simulink model "Model"  (R2024b)
settings: Solver=VariableStepAuto  StartTime=0.0  StopTime=30  MaxStep=0.001  RelTol=1e-4
PostLoadFcn:
  | SIM_setup
values from neighbouring files (symbols this model uses):
  A = 1.1    [RT14e_Parameters.m]    (also in RT15e_Parameters.m = 1.088; RT15evo_Parameters.m = 1.088; SIM_setup.m = 1.12)
  Aero_balance = 55    [RT14e_Parameters.m]    (also in RT15e_Parameters.m; RT15evo_Parameters.m; SIM_setup.m = 0.55)
  air_density = 1.29    [SIM_setup.m]
  Br_coef_of_friction_F = 0.33    [RT14e_Parameters.m]    (also in RT15e_Parameters.m; RT15evo_Parameters.m; SIM_setup.m = 0.25)
  Br_coef_of_friction_R = 0.33    [RT14e_Parameters.m]    (also in RT15e_Parameters.m; RT15evo_Parameters.m; SIM_setup.m = 0.25)
  Br_pistons_area_F = 3617.26/1e6    (= 0.00361726)    [RT14e_Parameters.m]    (also in RT15e_Parameters.m; RT15evo_Parameters.m; SIM_setup.m)
  Br_pistons_area_R = 2026.83/1e6    (= 0.00202683)    [RT14e_Parameters.m]    (also in RT15e_Parameters.m; RT15evo_Parameters.m; SIM_setup.m)
  Cd = 1.387    [SIM_setup.m]
  Cl = 3.299    [SIM_setup.m]
  CoG_z = 0.35    [RT14e_Parameters.m]    (also in RT15e_Parameters.m = 0.28495; RT15evo_Parameters.m = 0.28495; SIM_setup.m = 0.328)
  Default_Fz_F = g*(Mass*(Lr/Wheelbase))    [RT14e_Parameters.m]    (also in RT15e_Parameters.m; RT15evo_Parameters.m; SIM_setup.m = 608.22)
  Default_Fz_R = g*(Mass*(Lf/Wheelbase))    [RT14e_Parameters.m]    (also in RT15e_Parameters.m; RT15evo_Parameters.m; SIM_setup.m = 774.99)
  Effective_br_disk_r_F = 0.0905    [RT14e_Parameters.m]    (also in RT15e_Parameters.m; RT15evo_Parameters.m; SIM_setup.m)
  Effective_br_disk_r_R = 0.0895    [RT14e_Parameters.m]    (also in RT15e_Parameters.m; RT15evo_Parameters.m; SIM_setup.m)
  Fx = Data_Fx(2:end,3:end)    [RT14e_Parameters.m]    (also in RT15e_Parameters.m; RT15evo_Parameters.m; SIM_setup.m = Data_Fx(2:end,2:end))
  Fy = Data_Fy(2:end,3:end)    [RT14e_Parameters.m]    (also in RT15e_Parameters.m; RT15evo_Parameters.m; SIM_setup.m = Data_Fy(2:end,2:end))
  Fz = Data_Fy(2:end,2)    [RT14e_Parameters.m]    (also in RT15e_Parameters.m; RT15evo_Parameters.m; SIM_setup.m = Data_Fy(2:end,1))
  Half_track = 0.6    [SIM_setup.m]
  Iz_wehicle = 120    [RT14e_Parameters.m]    (also in RT15e_Parameters.m; RT15evo_Parameters.m; SIM_setup.m)
  Iz_wheel = 0.15    [RT14e_Parameters.m]    (also in RT15e_Parameters.m; RT15evo_Parameters.m; SIM_setup.m)
  Lateral_load_transfer_distribution = 0.55    [SIM_setup.m]
  Lf = Wheelbase - CoG_x    (= 0.77)    [RT14e_Parameters.m]    (also in RT15e_Parameters.m = 0.7504; RT15evo_Parameters.m = 0.7504; SIM_setup.m)
  Lr = Wheelbase - Lf    (= 0.755)    [RT14e_Parameters.m]    (also in RT15e_Parameters.m = 0.7746; RT15evo_Parameters.m = 0.7746; SIM_setup.m)
  Mass = Vehicle_mass + Driver_mass    (= 290)    [RT14e_Parameters.m]    (also in RT15e_Parameters.m = 265; RT15evo_Parameters.m; SIM_setup.m = 300)
  Max_Torque = 29.1    [SIM_setup.m]
  RB_torque_setting_1 = -2    [RT14e_Parameters.m]    (also in RT15e_Parameters.m; RT15evo_Parameters.m; SIM_setup.m)
  RB_torque_setting_10 = -20    [RT14e_Parameters.m]    (also in RT15e_Parameters.m; RT15evo_Parameters.m; SIM_setup.m)
  RB_torque_setting_2 = -4    [RT14e_Parameters.m]    (also in RT15e_Parameters.m; RT15evo_Parameters.m; SIM_setup.m)
  RB_torque_setting_3 = -6    [RT14e_Parameters.m]    (also in RT15e_Parameters.m; RT15evo_Parameters.m; SIM_setup.m)
  RB_torque_setting_4 = -8    [RT14e_Parameters.m]    (also in RT15e_Parameters.m; RT15evo_Parameters.m; SIM_setup.m)
  RB_torque_setting_5 = -10    [RT14e_Parameters.m]    (also in RT15e_Parameters.m; RT15evo_Parameters.m; SIM_setup.m)
  RB_torque_setting_6 = -12    [RT14e_Parameters.m]    (also in RT15e_Parameters.m; RT15evo_Parameters.m; SIM_setup.m)
  RB_torque_setting_7 = -14    [RT14e_Parameters.m]    (also in RT15e_Parameters.m; RT15evo_Parameters.m; SIM_setup.m)
  RB_torque_setting_8 = -16    [RT14e_Parameters.m]    (also in RT15e_Parameters.m; RT15evo_Parameters.m; SIM_setup.m)
  RB_torque_setting_9 = -18    [RT14e_Parameters.m]    (also in RT15e_Parameters.m; RT15evo_Parameters.m; SIM_setup.m)
  SA = Data_Fy(1,3:end)    [RT14e_Parameters.m]    (also in RT15e_Parameters.m; RT15evo_Parameters.m; SIM_setup.m = Data_Fy(1,2:end))
  SR = Data_Fx(1,3:end)    [RT14e_Parameters.m]    (also in RT15e_Parameters.m; RT15evo_Parameters.m; SIM_setup.m = Data_Fx(1,2:end))
  start_time = 182    [SIM_setup.m]
  start_velocity = Xsens_MTI_670_vel.Value(find(Xsens_MTI_670_vel.Time > start_time, 1)) * 1000 / 3600    [SIM_setup.m]
  Steering_angle_table = [0 9.9 19.9 30.14 40.57 51.05 61.29 70.87 79.38 91.9]    [SIM_setup.m]
  Steering_ratio_table = [3.25 3.24 3.23 3.20 3.16 3.10 3.04 2.97 2.90 2.77]    [SIM_setup.m]
  Tire_radius = 0.203    [RT14e_Parameters.m]    (also in RT15e_Parameters.m; RT15evo_Parameters.m; SIM_setup.m)
  Torque_limit_2 = Motor_maximum_torque*0.2    (= 5.82)    [RT14e_Parameters.m]    (also in RT15e_Parameters.m; RT15evo_Parameters.m; SIM_setup.m)
  Torque_limit_3 = Motor_maximum_torque*0.3    (= 8.73)    [RT14e_Parameters.m]    (also in RT15e_Parameters.m; RT15evo_Parameters.m; SIM_setup.m)
  Torque_limit_4 = Motor_maximum_torque*0.4    (= 11.64)    [RT14e_Parameters.m]    (also in RT15e_Parameters.m; RT15evo_Parameters.m; SIM_setup.m)
  Torque_limit_5 = Motor_maximum_torque*0.5    (= 14.55)    [RT14e_Parameters.m]    (also in RT15e_Parameters.m; RT15evo_Parameters.m; SIM_setup.m)
  Torque_limit_6 = Motor_maximum_torque*0.6    (= 17.46)    [RT14e_Parameters.m]    (also in RT15e_Parameters.m; RT15evo_Parameters.m; SIM_setup.m)
  Torque_limit_7 = Motor_maximum_torque*0.7    (= 20.37)    [RT14e_Parameters.m]    (also in RT15e_Parameters.m; RT15evo_Parameters.m; SIM_setup.m)
  Torque_limit_8 = Motor_maximum_torque*0.8    (= 23.28)    [RT14e_Parameters.m]    (also in RT15e_Parameters.m; RT15evo_Parameters.m; SIM_setup.m)
  Torque_limit_9 = 29.1    [RT14e_Parameters.m]    (also in RT15e_Parameters.m; RT15evo_Parameters.m; SIM_setup.m)
  Torque_limit_max = Motor_maximum_torque    (= 29.1)    [RT14e_Parameters.m]    (also in RT15e_Parameters.m; RT15evo_Parameters.m; SIM_setup.m)
  Torque_limit_min = Motor_maximum_torque*0.1    (= 2.91)    [RT14e_Parameters.m]    (also in RT15e_Parameters.m; RT15evo_Parameters.m; SIM_setup.m)
  Transmission_gear_ratio = 12.9    [SIM_setup.m]
  TV_RB_understeer_gradient_1 = -0.5    [RT14e_Parameters.m]    (also in RT15e_Parameters.m; RT15evo_Parameters.m; SIM_setup.m)
  TV_RB_understeer_gradient_10 = 0.005    [RT14e_Parameters.m]    (also in RT15e_Parameters.m; RT15evo_Parameters.m; SIM_setup.m)
  TV_RB_understeer_gradient_2 = -0.1    [RT14e_Parameters.m]    (also in RT15e_Parameters.m; RT15evo_Parameters.m; SIM_setup.m)
  TV_RB_understeer_gradient_3 = 0.08    [RT14e_Parameters.m]    (also in RT15e_Parameters.m; RT15evo_Parameters.m; SIM_setup.m)
  TV_RB_understeer_gradient_4 = 0.06    [RT14e_Parameters.m]    (also in RT15e_Parameters.m; RT15evo_Parameters.m; SIM_setup.m)
  TV_RB_understeer_gradient_5 = 0.05    [RT14e_Parameters.m]    (also in RT15e_Parameters.m; RT15evo_Parameters.m; SIM_setup.m)
  TV_RB_understeer_gradient_6 = 0.04    [RT14e_Parameters.m]    (also in RT15e_Parameters.m; RT15evo_Parameters.m; SIM_setup.m)
  TV_RB_understeer_gradient_7 = 0.03    [RT14e_Parameters.m]    (also in RT15e_Parameters.m; RT15evo_Parameters.m; SIM_setup.m)
  TV_RB_understeer_gradient_8 = 0.02    [RT14e_Parameters.m]    (also in RT15e_Parameters.m; RT15evo_Parameters.m; SIM_setup.m)
  TV_RB_understeer_gradient_9 = 0.01    [RT14e_Parameters.m]    (also in RT15e_Parameters.m; RT15evo_Parameters.m; SIM_setup.m)
  TV_understeer_gradient_1 = -0.5    [RT14e_Parameters.m]    (also in RT15e_Parameters.m; RT15evo_Parameters.m; SIM_setup.m)
  TV_understeer_gradient_10 = 0.002    [RT14e_Parameters.m]    (also in RT15e_Parameters.m; RT15evo_Parameters.m; SIM_setup.m)
  TV_understeer_gradient_2 = -0.1    [RT14e_Parameters.m]    (also in RT15e_Parameters.m; RT15evo_Parameters.m; SIM_setup.m)
  TV_understeer_gradient_3 = 0.06    [RT14e_Parameters.m]    (also in RT15e_Parameters.m; RT15evo_Parameters.m; SIM_setup.m)
  TV_understeer_gradient_4 = 0.05    [RT14e_Parameters.m]    (also in RT15e_Parameters.m; RT15evo_Parameters.m; SIM_setup.m)
  TV_understeer_gradient_5 = 0.04    [RT14e_Parameters.m]    (also in RT15e_Parameters.m; RT15evo_Parameters.m; SIM_setup.m)
  TV_understeer_gradient_6 = 0.03    [RT14e_Parameters.m]    (also in RT15e_Parameters.m; RT15evo_Parameters.m; SIM_setup.m)
  TV_understeer_gradient_7 = 0.02    [RT14e_Parameters.m]    (also in RT15e_Parameters.m; RT15evo_Parameters.m; SIM_setup.m)
  TV_understeer_gradient_8 = 0.01    [RT14e_Parameters.m]    (also in RT15e_Parameters.m; RT15evo_Parameters.m; SIM_setup.m)
  TV_understeer_gradient_9 = 0.005    [RT14e_Parameters.m]    (also in RT15e_Parameters.m; RT15evo_Parameters.m; SIM_setup.m)
  Wheel_base = 1.525    [SIM_setup.m]
  Wheel_rolling_resistance = 0.055    [RT14e_Parameters.m]    (also in RT15e_Parameters.m; RT15evo_Parameters.m; SIM_setup.m)
undefined symbols (not defined in the file or in its folder): Actual_Torque_Value_RL, Actual_Torque_Value_RR, aero_balance, APPS, Brake_Pressure_Front, Brake_Pressure_Rear, lateral_load_transfer_distribution, Steering_position, tire_radius, wheel_base, Xsens_MTI_670_accX, Xsens_MTI_670_accY, Xsens_MTI_670_gyrZ, Xsens_MTI_670_vel, Xsens_Yaw_Rate__deg_s_
libraries: simulink x20, simulink_extras x7, dspstat3 x4, slpidlib x1, slrealtimeloglib x1
(part 2 of 4)

== system Model/Drivetrain/Braking_Torque/Braking_Torque_Front ==
  Brake_Pressure [bar] : Inport
  Gain : Gain  Gain=1e5
  Gain1 : Gain  Gain=Effective_br_disk_r_F
  Product : Product  Inputs=3
  coefficient of friction : Constant  Value=Br_coef_of_friction_F
  piston area : Constant  Value=Br_pistons_area_F
  Braking torque [Nm] : Outport
  wires:
  Brake_Pressure [bar]/1 -> Gain/1  "[bar]"
  Gain/1 -> Product/1  "[Pa]"
  coefficient of friction/1 -> Product/2
  piston area/1 -> Product/3
  Product/1 -> Gain1/1  "Braking force [N]"
  Gain1/1 -> Braking torque [Nm]/1  "Braking torque [Nm]"

== system Model/Drivetrain/Braking_Torque/Braking_Torque_Rear ==
  Brake_Pressure [bar] : Inport
  Gain1 : Gain  Gain=1e5
  Gain2 : Gain  Gain=Effective_br_disk_r_R
  Product2 : Product  Inputs=3
  coefficient of friction : Constant  Value=Br_coef_of_friction_R
  piston area : Constant  Value=Br_pistons_area_R
  Braking_Torque [Nm] : Outport
  wires:
  Product2/1 -> Gain2/1  "Braking_Force [N]"
  piston area/1 -> Product2/3
  Gain2/1 -> Braking_Torque [Nm]/1  "Braking_Torque [Nm]"
  Gain1/1 -> Product2/1  "[Pa]"
  coefficient of friction/1 -> Product2/2
  Brake_Pressure [bar]/1 -> Gain1/1

== system Model/Drivetrain/Engine_Power/Engine_RL ==
  Wheel_Angular_Speed : Inport
  Engine_Torque : Inport  Port=2
  Gain : Gain  Gain=60/2*pi
  Gain1 : Gain  Gain=1/3.6e7
  Integrator : Integrator
  Product : Product
  Energy Used [kWh] : Outport
  wires:
  Gain/1 -> Product/1  "Wheel_Angular_Speed [rot/min]"
  Gain1/1 -> Energy Used [kWh]/1  "Energy_Used [kWh]"
  Integrator/1 -> Gain1/1  "Energy [J]"
  Product/1 -> Integrator/1  "Motor_Power [W]"
  Wheel_Angular_Speed/1 -> Gain/1
  Engine_Torque/1 -> Product/2

== system Model/Drivetrain/Engine_Power/Engine_RR ==
  Wheel_Angular_Speed : Inport
  Engine_Torque : Inport  Port=2
  Gain : Gain  Gain=60/2*pi
  Gain1 : Gain  Gain=1/3.6e7
  Integrator : Integrator
  Product : Product
  Energy Used [kWh] : Outport
  wires:
  Gain/1 -> Product/1  "Wheel_Angular_Speed [rot/min]"
  Gain1/1 -> Energy Used [kWh]/1  "Energy_Used [kWh]"
  Integrator/1 -> Gain1/1  "Energy [J]"
  Product/1 -> Integrator/1  "Motor_Power [W]"
  Wheel_Angular_Speed/1 -> Gain/1
  Engine_Torque/1 -> Product/2

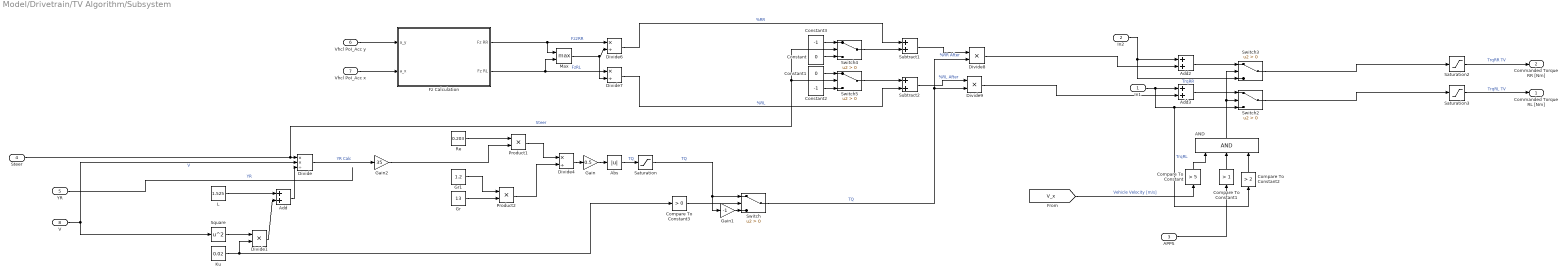
== system Model/Drivetrain/TV Algorithm/Subsystem ==
  In1 : Inport
  In2 : Inport  Port=2
  APPS : Inport  Port=3
  Steer : Inport  Port=4
  YR : Inport  Port=5
  Vhcl PoI_Acc y : Inport  Port=6
  Vhcl PoI_Acc x : Inport  Port=7
  V : Inport  Port=8
  AND : Logic  Inputs=3  IconShape=distinctive  AllPortsSameDT=off  OutDataTypeStr=boolean
  Abs : Abs  SaturateOnIntegerOverflow=off
  Add : Sum
  Add2 : Sum
  Add3 : Sum
  Compare To Constant : simulink/Logic and Bit Operations/Compare To Constant  relop=>  const=5  OutDataTypeStr=boolean
  Compare To Constant1 : simulink/Logic and Bit Operations/Compare To Constant  relop=>  const=1  OutDataTypeStr=boolean
  Compare To Constant2 : simulink/Logic and Bit Operations/Compare To Constant  relop=>  const=2  OutDataTypeStr=boolean
  Compare To Constant3 : simulink/Logic and Bit Operations/Compare To Constant  relop=>  const=0  OutDataTypeStr=boolean
  Constant : Constant  Value=0
  Constant1 : Constant  Value=0
  Constant2 : Constant  Value=-1
  Constant3 : Constant  Value=-1
  Divide : Product  Inputs=**/
  Divide1 : Product  Inputs=**
  Divide4 : Product  Inputs=*/
  Divide6 : Product  Inputs=*/
  Divide7 : Product  Inputs=*/
  Divide8 : Product  Inputs=**
  Divide9 : Product  Inputs=**
  Fz Calculation : Subsystem
  Gain : Gain  Gain=0.5
  Gain1 : Gain  Gain=-1
  Gain2 : Gain  Gain=35
  Gr : Constant  Value=13
  Gr1 : Constant  Value=1.2
  Ku : Constant  Value=0.02
  L : Constant  Value=1.525
  Max : MinMax  Function=max  Inputs=2
  Product1 : Product
  Product2 : Product
  Re : Constant  Value=0.203
  Saturation : Saturate  UpperLimit=8  LowerLimit=0
  Saturation2 : Saturate  UpperLimit=Max_Torque  LowerLimit=0
  Saturation3 : Saturate  UpperLimit=Max_Torque  LowerLimit=0
  Square : Math  Operator=square
  Subtract1 : Sum
  Subtract2 : Sum
  Switch{,2..5} (5 alike) : Switch  Criteria=u2 > Threshold  SaturateOnIntegerOverflow=off  InputSameDT=off
  Commanded Torque RL [Nm] : Outport
  Commanded Torque RR [Nm] : Outport  Port=2
  wires:
  Max/1 -> Divide7/2, Divide6/2
  Divide9/1 -> Add3/2
  L/1 -> Add/1
  Steer/1 -> Switch4/2, Switch5/2, Divide/1  "Steer"
  In1/1 -> Compare To Constant2/1, Switch2/3, Add3/1  "TrqRL"
  Vhcl PoI_Acc y/1 -> Fz Calculation/1(a_y)
  Divide8/1 -> Add2/2
  Divide6/1 -> Subtract1/1  "%RR"
  In2/1 -> Switch3/3, Add2/1  "TrqRR"
  Vhcl PoI_Acc x/1 -> Fz Calculation/2(a_x)
  Divide4/1 -> Gain/1
  Add3/1 -> Switch2/1
  Divide7/1 -> Subtract2/2  "%RL"
  Divide1/1 -> Add/2
  Ku/1 -> Compare To Constant3/1, Divide1/2
  Add/1 -> Divide/3
  Divide/1 -> Gain2/1  "YR Calc"
  Fz Calculation/2(Fz RL) -> Max/2, Divide7/1  "FzRL"
  Square/1 -> Divide1/1
  Saturation2/1 -> Commanded Torque RR [Nm]/1  "TrqRR TV"
  Saturation3/1 -> Commanded Torque RL [Nm]/1  "TrqRL TV"
  Re/1 -> Product1/1
  Product1/1 -> Divide4/1
  Gr/1 -> Product2/2
  Gain2/1 -> Product1/2
  Switch/1 -> Divide8/2, Divide9/2  "TQ"
  YR/1 -> ?  "YR"
  Gr1/1 -> Product2/1
  Product2/1 -> Divide4/2
  V/1 -> Square/1, Divide/2  "V"
  Gain/1 -> Abs/1
  Add2/1 -> Switch3/1
  [V_x] -> Compare To Constant/1  "Vehicle Velocity [m/s]"
  Compare To Constant/1 -> AND/1
  Compare To Constant1/1 -> AND/2
  APPS/1 -> Compare To Constant1/1
  AND/1 -> Switch2/2, Switch3/2
  Abs/1 -> Saturation/1  "TQ"
  Subtract1/1 -> Divide8/1  "%RR After"
  Subtract2/1 -> Divide9/1  "%RL After"
  Constant2/1 -> Switch5/3
  Switch4/1 -> Subtract1/2
  Switch5/1 -> Subtract2/1
  Constant/1 -> Switch4/3
  Constant1/1 -> Switch5/1
  Constant3/1 -> Switch4/1
  Compare To Constant2/1 -> AND/3
  Switch3/1 -> Saturation2/1
  Switch2/1 -> Saturation3/1
  Compare To Constant3/1 -> Switch/2
  Saturation/1 -> Switch/1, Gain1/1  "TQ"
  Gain1/1 -> Switch/3
  Fz Calculation/1(Fz RR) -> Max/1, Divide6/1  "Fz2RR"

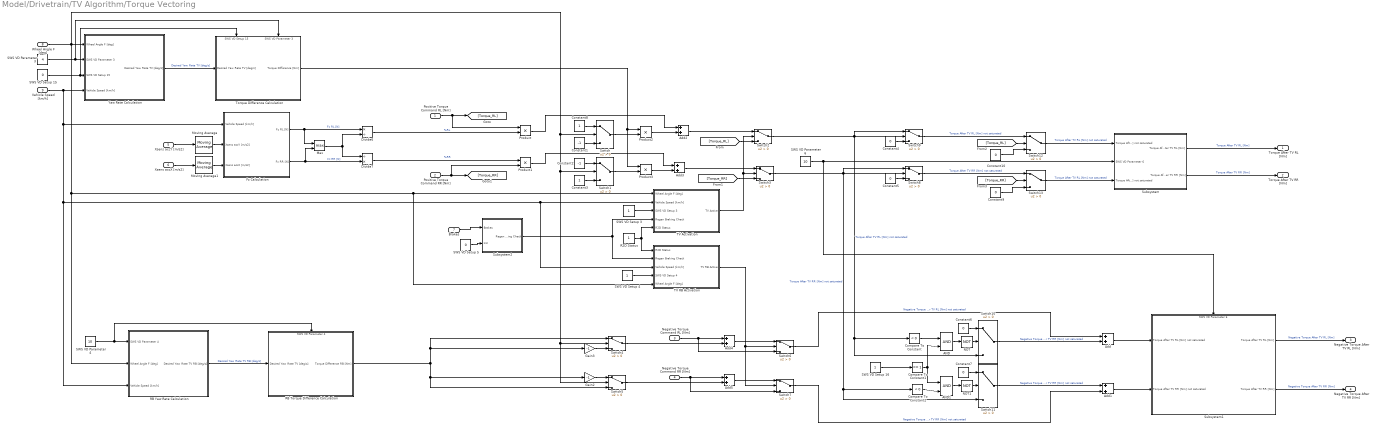
== system Model/Drivetrain/TV Algorithm/Torque Vectoring ==
  Positive Torque Command RL [Nm] : Inport
  Positive Torque Command RR [Nm] : Inport  Port=2
  Negative Torque Command RL [Nm] : Inport  Port=3
  Negative Torque Command RR [Nm] : Inport  Port=4
  Xsens accY [m/s2] : Inport  Port=5
  Xsens accX [m/s2] : Inport  Port=6
  Brakes : Inport  Port=7
  Wheel Angle F [deg] : Inport  Port=8
  Vehicle Speed [km/h] : Inport  Port=9
  AND : Logic  IconShape=distinctive  AllPortsSameDT=off  OutDataTypeStr=boolean
  AND1 : Logic  IconShape=distinctive  AllPortsSameDT=off  OutDataTypeStr=boolean
  Add{,1..5} (6 alike) : Sum
  Compare To Constant : simulink/Logic and Bit Operations/Compare To Constant  relop=<  const=0  OutDataTypeStr=boolean
  Compare To Constant1 : simulink/Logic and Bit Operations/Compare To Constant  relop===  const=1  OutDataTypeStr=boolean
  Compare To Constant2 : simulink/Logic and Bit Operations/Compare To Constant  relop=<  const=0  OutDataTypeStr=boolean
  Constant1 : Constant  Value=-1
  Constant{4..7,9..10} (6 alike) : Constant  Value=0
  Constant2 : Constant  Value=-1
  Constant3 : Constant
  Constant8 : Constant
  Divide6 : Product  Inputs=*/
  Divide7 : Product  Inputs=/*
  Fz Calculation : Subsystem
  Gain2 : Gain  Gain=-1
  Gain3 : Gain  Gain=-1
  Max : MinMax  Function=max  Inputs=2
  Moving Average : dspstat3/Moving Average  Method=Sliding window  ForgettingFactorPort=off  SpecifyWindowLength=on  WindowLength=4  OverlapLength=3  AllowArbitraryInputLength=off  ForgettingFactor=0.9  SimulateUsing=Code generation
  Moving Average1 : dspstat3/Moving Average  Method=Sliding window  ForgettingFactorPort=off  SpecifyWindowLength=on  WindowLength=4  OverlapLength=3  AllowArbitraryInputLength=off  ForgettingFactor=0.9  SimulateUsing=Code generation
  NOT : Logic  Operator=NOT  IconShape=distinctive  AllPortsSameDT=off  OutDataTypeStr=boolean
  NOT1 : Logic  Operator=NOT  IconShape=distinctive  AllPortsSameDT=off  OutDataTypeStr=boolean
  Product{,1..3} (4 alike) : Product
  R2D Status : Constant
  RB Torque Difference Calculation : Subsystem
      settings: PortSchema="{\"entries\":[{\"content\":{\"sides\":[{\"content\":{\"connectorIds\":[\"In1\"]},\"type\":\"ConnectorPlacement.EquallySpacedRectSide\",\"uuid\":\"fa4973ad-a32f-4095-ab0b-cea383016739\"},{\"content\":{\"connectorIds\":[\"Out1\"],\"side\":\"RIGHT\"},\"type\":\"ConnectorPlacement.EquallySpacedRectSide\",\"uuid\":\"939e1308-df81-4bd9-8a82-65ce288053d3\"},{\"content\":{\"connectorIds\":[\"In2\"],\"side\":\"TOP\"},\"type\":\"ConnectorPlacement.EquallySpacedRectSide\",\"uuid\":\"fc465ebf-5b67-4318-901e-ca5dd36e3a85\"}]},\"type\":\"ConnectorPlacement.EquallySpacedConnector\",\"uuid\":\"4f087700-9ed6-4341-833d-4cc93a86ad38\"}],\"packageUris\":[\"http://schema.mathworks.com/mf0/Connector/R2020b\"],\"version\":\"1.0\"}"
  RB Yaw Rate Calculation : Subsystem
  SWS VD Parameter 3 : Constant  Value=4
  SWS VD Parameter 4 : Constant  Value=10
  SWS VD Parameter 6 : Constant  Value=10
  SWS VD Setup 15 : Constant  Value=0
  SWS VD Setup 16 : Constant
  SWS VD Setup 3 : Constant
  SWS VD Setup 4 : Constant
  SWS VD Setup 5 : Constant  Value=0
  Subsystem : Subsystem
  Subsystem1 : Subsystem
      settings: PortSchema="{\"entries\":[{\"content\":{\"sides\":[{\"content\":{\"connectorIds\":[\"In1\",\"In2\"]},\"type\":\"ConnectorPlacement.EquallySpacedRectSide\",\"uuid\":\"3056adb4-125a-41ff-b8f3-94632bed0e59\"},{\"content\":{\"connectorIds\":[\"Out1\",\"Out2\"],\"side\":\"RIGHT\"},\"type\":\"ConnectorPlacement.EquallySpacedRectSide\",\"uuid\":\"828b5026-b9f0-47a0-9847-e54771aaad3f\"},{\"content\":{\"connectorIds\":[\"In3\"],\"side\":\"TOP\"},\"type\":\"ConnectorPlacement.EquallySpacedRectSide\",\"uuid\":\"5565ffc5-94d3-407e-898e-a464d97134f1\"}]},\"type\":\"ConnectorPlacement.EquallySpacedConnector\",\"uuid\":\"ef74bfd7-20f4-4a9c-8af2-e6f991f2b9d8\"}],\"packageUris\":[\"http://schema.mathworks.com/mf0/Connector/R2020b\"],\"version\":\"1.0\"}"
  Subsystem2 : Subsystem
  Switch{,1..13} (14 alike) : Switch  Criteria=u2 > Threshold  SaturateOnIntegerOverflow=off  InputSameDT=off
  TV Activation : Subsystem
  TV RB Activation : Subsystem
  Torque Difference Calculation : Subsystem
      settings: PortSchema="{\"entries\":[{\"content\":{\"sides\":[{\"content\":{\"connectorIds\":[\"In1\"]},\"type\":\"ConnectorPlacement.EquallySpacedRectSide\",\"uuid\":\"fa4973ad-a32f-4095-ab0b-cea383016739\"},{\"content\":{\"connectorIds\":[\"Out1\"],\"side\":\"RIGHT\"},\"type\":\"ConnectorPlacement.EquallySpacedRectSide\",\"uuid\":\"939e1308-df81-4bd9-8a82-65ce288053d3\"},{\"content\":{\"connectorIds\":[\"In2\",\"In3\"],\"side\":\"TOP\"},\"type\":\"ConnectorPlacement.EquallySpacedRectSide\",\"uuid\":\"fc465ebf-5b67-4318-901e-ca5dd36e3a85\"}]},\"type\":\"ConnectorPlacement.EquallySpacedConnector\",\"uuid\":\"4f087700-9ed6-4341-833d-4cc93a86ad38\"}],\"packageUris\":[\"http://schema.mathworks.com/mf0/Connector/R2020b\"],\"version\":\"1.0\"}"
  Yaw Rate Calculation : Subsystem
  Torque After TV RL [Nm] : Outport
  Torque After TV RR [Nm] : Outport  Port=2
  Negative Torque After TV RL [Nm] : Outport  Port=3
  Negative Torque After TV RR [Nm] : Outport  Port=4
  wires:
  Moving Average1/1 -> Fz Calculation/3(Xsens accX [m/s2])
  R2D Status/1 -> TV RB Activation/1(R2D Status), TV Activation/5(R2D Status)
  TV Activation/1(TV Active) -> Switch2/2, Switch3/2
  Subsystem/2(Torque After TV RR [Nm]) -> Torque After TV RR [Nm]/1  "Torque After TV RR [Nm]"
  Yaw Rate Calculation/1(Desired Yaw Rate TV [deg/s]) -> Torque Difference Calculation/1(Desired Yaw Rate TV [deg/s])  "Desired Yaw Rate TV [deg/s]"
  Fz Calculation/1(Fz RL [N]) -> Divide6/1, Max/1  "Fz RL [N]"
  Xsens accY [m/s2]/1 -> Moving Average/1
  Subsystem/1(Torque After TV RL [Nm]) -> Torque After TV RL [Nm]/1  "Torque After TV RL [Nm]"
  SWS VD Setup 3/1 -> TV Activation/3(SWS VD Setup 3)
  Divide6/1 -> Product/2  "%RL"
  Switch3/1 -> Switch8/2, Compare To Constant2/1, Switch11/3, Switch8/1  "Torque After TV RR [Nm] not saturated"
  Wheel Angle F [deg]/1 -> RB Yaw Rate Calculation/2(Wheel Angle F [deg]), TV RB Activation/5(Wheel Angle F [deg]), TV Activation/1(Wheel Angle F [deg]), Switch5/2, Switch4/2, Switch1/2, Switch/2, Yaw Rate Calculation/1(Wheel Angle F [deg])
  Xsens accX [m/s2]/1 -> Moving Average1/1
  SWS VD Parameter 3/1 -> Yaw Rate Calculation/2(SWS VD Parameter 3), Torque Difference Calculation/3(SWS VD Parameter 3)
  Divide7/1 -> Product1/1  "%RR"
  Switch2/1 -> Compare To Constant/1, Switch10/3, Switch9/1, Switch9/2  "Torque After TV RL [Nm] not saturated"
  Max/1 -> Divide6/2, Divide7/1
  Vehicle Speed [km/h]/1 -> Fz Calculation/1(Vehicle Speed [km/h]), TV RB Activation/3(Vehicle Speed [km/h]), TV Activation/2(Vehicle Speed [km/h]), RB Yaw Rate Calculation/3(Vehicle Speed [km/h]), Yaw Rate Calculation/4(Vehicle Speed [km/h])
  Fz Calculation/2(Fz RR [N]) -> Max/2, Divide7/2  "Fz RR [N]"
  Moving Average/1 -> Fz Calculation/2(Xsens accY [m/s2])
  SWS VD Parameter 6/1 -> Subsystem1/3(SWS VD Parameter 6), Subsystem/2(SWS VD Parameter 6)
  Torque Difference Calculation/1(Torque Difference [Nm]) -> Product3/1, Product2/1
  Negative Torque Command RL [Nm]/1 -> Switch6/3, Add4/1
  Switch4/1 -> Add4/2
  Switch5/1 -> Add5/2
  Negative Torque Command RR [Nm]/1 -> Add5/1, Switch7/3
  Add4/1 -> Switch6/1
  TV RB Activation/1(TV RB Active) -> Switch6/2, Switch7/2
  Add5/1 -> Switch7/1
  SWS VD Setup 4/1 -> TV RB Activation/4(SWS VD Setup 4)
  Subsystem1/1(Torque After TV RL [Nm]) -> Negative Torque After TV RL [Nm]/1  "Negative Torque After TV RL [Nm]"
  Subsystem1/2(Torque After TV RR [Nm]) -> Negative Torque After TV RR [Nm]/1  "Negative Torque After TV RR [Nm]"
  Gain2/1 -> Switch5/1
  Gain3/1 -> Switch4/3
  Positive Torque Command RL [Nm]/1 -> [Torque_RL], Product/1
  Positive Torque Command RR [Nm]/1 -> [Torque_RR], Product1/2
  Constant8/1 -> Switch/1
  Constant1/1 -> Switch/3
  Constant2/1 -> Switch1/1
  Constant3/1 -> Switch1/3
  Switch/1 -> Product2/2
  Switch1/1 -> Product3/2
  [Torque_RR] -> Switch3/3
  [Torque_RL] -> Switch2/3
  Constant4/1 -> Switch9/3
  Constant5/1 -> Switch8/3
  Switch9/1 -> Switch12/1  "Torque After TV RL [Nm] not saturated"
  Switch8/1 -> Switch13/1  "Torque After TV RR [Nm] not saturated"
  Constant6/1 -> Switch10/1
  Add/1 -> Subsystem1/1(Torque After TV RL [Nm] not saturated)
  Constant7/1 -> Switch11/1
  Add1/1 -> Subsystem1/2(Torque After TV RR [Nm] not saturated)
  Add2/1 -> Switch2/1
  Product2/1 -> Add2/2
  Product/1 -> Add2/1
  Product1/1 -> Add3/1
  Product3/1 -> Add3/2
  Add3/1 -> Switch3/1
  SWS VD Setup 15/1 -> Torque Difference Calculation/2(SWS VD Setup 15), Yaw Rate Calculation/3(SWS VD Setup 15)
  [Torque_RL] -> Switch12/2
  [Torque_RR] -> Switch13/2
  Constant9/1 -> Switch13/3
  Constant10/1 -> Switch12/3
  Switch12/1 -> Subsystem/1(Torque After TV RL [Nm] not saturated)  "Torque After TV RL [Nm] not saturated"
  Switch13/1 -> Subsystem/3(Torque After TV RR [Nm] not saturated)  "Torque After TV RL [Nm] not saturated"
  RB Yaw Rate Calculation/1(Desired Yaw Rate TV RB [deg/s]) -> RB Torque Difference Calculation/1(Desired Yaw Rate TV [deg/s])  "Desired Yaw Rate TV RB [deg/s]"
  RB Torque Difference Calculation/1(Torque Difference RB [Nm]) -> Switch4/1, Gain3/1, Switch5/3, Gain2/1
  Subsystem2/1(Regen Braking Check) -> TV Activation/4(Regen Braking Check), TV RB Activation/2(Regen Braking Check)
  SWS VD Parameter 4/1 -> RB Torque Difference Calculation/2(SWS VD Parameter 4), RB Yaw Rate Calculation/1(SWS VD Parameter 4)
  Compare To Constant/1 -> AND/1
  Compare To Constant1/1 -> AND/2, AND1/1
  SWS VD Setup 16/1 -> Compare To Constant1/1
  Switch11/1 -> Add1/1  "Negative Torque After TV RR [Nm] not saturated"
  Switch10/1 -> Add/2  "Negative Torque After TV RR [Nm] not saturated"
  AND/1 -> NOT/1
  AND1/1 -> NOT1/1
  Compare To Constant2/1 -> AND1/2
  Switch6/1 -> Add/1  "Negative Torque After TV RL [Nm] not saturated"
  Switch7/1 -> Add1/2  "Negative Torque After TV RR [Nm] not saturated"
  NOT/1 -> Switch10/2
  NOT1/1 -> Switch11/2
  SWS VD Setup 5/1 -> Subsystem2/2(In3)
  Brakes/1 -> Subsystem2/1(Brakes)

== system Model/Tires /Subsystem1/Slip Angle ==
  X_Velocity [m/s] : Inport
  Y_Velocity [m/s] : Inport  Port=2
  Yaw_Rate [rad/s] : Inport  Port=3
  Steering_Angle [rad] : Inport  Port=4
  Demux2 : Demux  Outputs=2
  Mux2 : Mux
  Slip Angle FL : Subsystem
  Slip Angle FR : Subsystem
  Slip Angle RL : Subsystem
  Slip Angle RR : Subsystem
  Slip_Angle [rad] : Outport
  wires:
  Y_Velocity [m/s]/1 -> Slip Angle FL/1(Y_Velocity), Slip Angle FR/1(Y_Velocity), Slip Angle RR/1(Y_Velocity), Slip Angle RL/1(Y_Velocity)
  Yaw_Rate [rad/s]/1 -> Slip Angle FL/2(Yaw_Rate), Slip Angle RR/2(Yaw_Rate), Slip Angle RL/2(Yaw_Rate), Slip Angle FR/2(Yaw_Rate)
  X_Velocity [m/s]/1 -> Slip Angle FL/3(X_Velocity), Slip Angle FR/3(X_Velocity), Slip Angle RR/3(X_Velocity), Slip Angle RL/3(X_Velocity)
  Steering_Angle [rad]/1 -> Demux2/1
  Demux2/2 -> Slip Angle FR/4(Steering_Angle_FR)
  Demux2/1 -> Slip Angle FL/4(Steering_Angle_FL)
  Mux2/1 -> Slip_Angle [rad]/1
  Slip Angle FL/1(Slip_Angle_FL) -> Mux2/1
  Slip Angle FR/1(Slip_Angle_FR) -> Mux2/2
  Slip Angle RL/1(Slip_Angle_RL) -> Mux2/3
  Slip Angle RR/1(Slip_Angle_RR) -> Mux2/4

== system Model/Tires /Subsystem1/Slip Ratio ==
  Wheels_Angular_Speed [rad/s] : Inport
  X_Velocity [m/s] : Inport  Port=2
  Bus Selector : BusSelector  OutputSignals=FL,FR,RL,RR
  Mux : Mux
  Slip ratio FL : Subsystem
  Slip ratio FR : Subsystem
  Slip ratio RL : Subsystem
  Slip ratio RR : Subsystem
  Slip_Ratio : Outport
  wires:
  Wheels_Angular_Speed [rad/s]/1 -> Bus Selector/1
  Mux/1 -> Slip_Ratio/1
  Bus Selector/1 -> Slip ratio FL/1(Wheel_Angular_Speed_FR [rad/s])  "<FL>"
  Bus Selector/2 -> Slip ratio FR/1(Wheel_Angular_Speed_FL [rad/s])  "<FR>"
  Bus Selector/3 -> Slip ratio RL/1(Wheel_Angular_Speed_RL [rad/s])  "<RL>"
  Bus Selector/4 -> Slip ratio RR/1(Wheel_Angular_Speed_RR [rad/s])  "<RR>"
  Slip ratio FL/1(Slip_Ratio_FL) -> Mux/1
  Slip ratio FR/1(Slip _Ratio_FR) -> Mux/2
  Slip ratio RL/1(Slip_Ratio_RL) -> Mux/3
  Slip ratio RR/1(Slip_Ratio_RR) -> Mux/4
  X_Velocity [m/s]/1 -> Slip ratio RR/2(X_Velocity [m/s]), Slip ratio RL/2(X_Velocity [m/s]), Slip ratio FR/2(X_Velocity [m/s]), Slip ratio FL/2(X_Velocity [m/s])

== system Model/Tires /Subsystem1/wheel_speed ==
  Torque : Inport
  Fx : Inport  Port=2
  Fz : Inport  Port=3
  Bus Creator : BusCreator  Inputs=4
  Bus Selector : BusSelector  OutputSignals=FL,FR,RL,RR
  Demux : Demux
  FL_Angular_Speed : Subsystem
  FR_Angular_Speed : Subsystem
  Mux : Mux
  RL_Angular_Speed : Subsystem
  RR_Angular_Speed : Subsystem
  Subsystem2 : Subsystem
  Wheels_Angular_Speed [rad/s] : Outport
  wires:
  Fx/1 -> Bus Selector/1
  Bus Creator/1 -> Wheels_Angular_Speed [rad/s]/1  "Wheels_Angular_Speed [rad/s]"
  FR_Angular_Speed/1(Wheel_Angular_Speed_FR [rad/s]) -> Bus Creator/2  "FR"
  FL_Angular_Speed/1(Wheel_Angular_Speed_FL [rad/s]) -> Bus Creator/1  "FL"
  RL_Angular_Speed/1(Wheel_Angular_Speed_RL [rad/s]) -> Bus Creator/3  "RL"
  RR_Angular_Speed/1(Wheel_Angular_Speed_RR [rad/s]) -> Bus Creator/4  "RR"
  Bus Selector/1 -> Mux/1  "<FL>"
  Bus Selector/2 -> Mux/2  "<FR>"
  Demux/4 -> RR_Angular_Speed/3(Fx)
  Demux/3 -> RL_Angular_Speed/3(Fx)
  Demux/2 -> FR_Angular_Speed/3(Fx)
  Demux/1 -> FL_Angular_Speed/3(Fx)
  Bus Selector/3 -> Mux/3  "<RL>"
  Bus Selector/4 -> Mux/4  "<RR>"
  Fz/1 -> Subsystem2/1(Fz)
  Subsystem2/1(Rolling_Resistance) -> FL_Angular_Speed/2(Rolling_Resistance), FR_Angular_Speed/2(Rolling_Resistance), RR_Angular_Speed/2(Rolling_Resistance), RL_Angular_Speed/2(Rolling_Resistance)
  Mux/1 -> Demux/1
  Torque/1 -> RR_Angular_Speed/1(Torque), RL_Angular_Speed/1(Torque), FR_Angular_Speed/1(Torque), FL_Angular_Speed/1(Torque)

== system Model/Drivetrain/TV Algorithm/Subsystem/Fz Calculation ==
  a_y : Inport
  a_x : Inport  Port=2
  Add : Sum
  Add1 : Sum
  Fz RL Calculation : Subsystem
  Fz RR Calculation : Subsystem
  Gain : Gain  Gain=0.5
  Gain1 : Gain  Gain=air_density
  Gain2 : Gain  Gain=1/2
  Gain3 : Gain  Gain=Cl
  Gain4 : Gain  Gain=A
  Gain5 : Gain  Gain=aero_balance
  Square : Math  Operator=square
  Fz RR : Outport
  Fz RL : Outport  Port=2
  wires:
  a_x/1 -> Fz RL Calculation/2(a_x), Fz RR Calculation/2(a_x)  "ax"
  a_y/1 -> Fz RL Calculation/1(a_y), Fz RR Calculation/1(a_y)  "ay"
  Gain2/1 -> Gain3/1
  Square/1 -> Gain4/1
  Gain3/1 -> Gain5/1  "Downforce [N]"
  Gain1/1 -> Gain2/1
  Gain4/1 -> Gain1/1
  [V_x] -> Square/1  "Vehicle Velocity [m/s]"
  Add/1 -> Fz RR/1  "Fz RR"
  Fz RR Calculation/1(Fz RR) -> Add/2
  Gain5/1 -> Gain/1  "Downforce Rear"
  Gain/1 -> Add1/1, Add/1
  Fz RL Calculation/1(Fz RL) -> Add1/2
  Add1/1 -> Fz RL/1  "Fz RL"

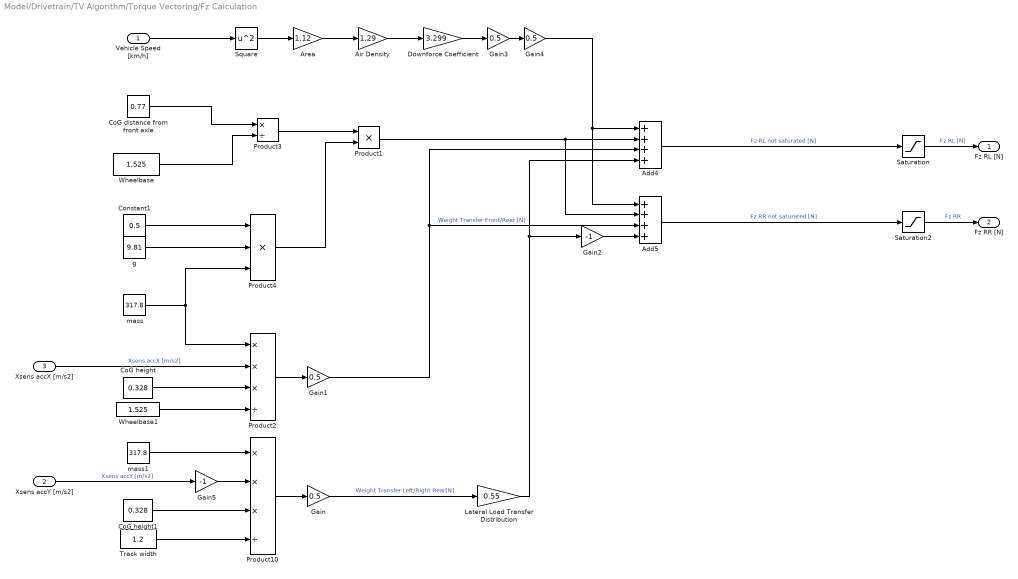
== system Model/Drivetrain/TV Algorithm/Torque Vectoring/Fz Calculation ==
  Vehicle Speed [km/h] : Inport
  Xsens accY [m/s2] : Inport  Port=2
  Xsens accX [m/s2] : Inport  Port=3
  Add4 : Sum  Inputs=++++
  Add5 : Sum  Inputs=++++
  Air Density : Gain  Gain=1.29
  Area : Gain  Gain=1.12
  CoG distance from front axle : Constant  Value=0.77
  CoG height : Constant  Value=0.328
  CoG height1 : Constant  Value=0.328
  Constant1 : Constant  Value=0.5
  Downforce Coefficient : Gain  Gain=3.299
  Gain{,1,3..4} (4 alike) : Gain  Gain=0.5
  Gain2 : Gain  Gain=-1
  Gain5 : Gain  Gain=-1
  Lateral Load Transfer Distribution : Gain  Gain=0.55
  Product1 : Product
  Product10 : Product  Inputs=***/
  Product2 : Product  Inputs=***/
  Product3 : Product  Inputs=*/
  Product4 : Product  Inputs=3
  Saturation : Saturate  UpperLimit=10000  LowerLimit=0
  Saturation2 : Saturate  UpperLimit=10000  LowerLimit=0
  Square : Math  Operator=square
  Track width : Constant  Value=1.2
  Wheelbase : Constant  Value=1.525
  Wheelbase1 : Constant  Value=1.525
  g : Constant  Value=9.81
  mass : Constant  Value=317.8
  mass1 : Constant  Value=317.8
  Fz RL [N] : Outport
  Fz RR [N] : Outport  Port=2
  wires:
  Xsens accX [m/s2]/1 -> Product2/2  "Xsens accX [m/s2]"
  Xsens accY [m/s2]/1 -> Gain5/1  "Xsens accY [m/s2]"
  Add5/1 -> Saturation2/1  "Fz RR not saturated [N]"
  Saturation2/1 -> Fz RR [N]/1  "Fz RR"
  Saturation/1 -> Fz RL [N]/1  "Fz RL [N]"
  Add4/1 -> Saturation/1  "Fz RL not saturated [N]"
  Product2/1 -> Gain1/1
  Product3/1 -> Product1/1
  CoG distance from front axle/1 -> Product3/1
  Wheelbase1/1 -> Product2/4
  CoG height/1 -> Product2/3
  mass/1 -> Product4/3, Product2/1
  Product10/1 -> Gain/1
  Constant1/1 -> Product4/1
  Track width/1 -> Product10/4
  g/1 -> Product4/2
  Product4/1 -> Product1/2
  Wheelbase/1 -> Product3/2
  CoG height1/1 -> Product10/3
  mass1/1 -> Product10/1
  Gain/1 -> Lateral Load Transfer Distribution/1  "Weight Transfer Left/Right Rear[N]"
  Gain1/1 -> Add4/3, Add5/3  "Weight Transfer Front/Rear [N]"
  Lateral Load Transfer Distribution/1 -> Add4/4, Gain2/1
  Product1/1 -> Add4/2, Add5/2
  Gain2/1 -> Add5/4
  Vehicle Speed [km/h]/1 -> Square/1
  Square/1 -> Area/1
  Area/1 -> Air Density/1
  Air Density/1 -> Downforce Coefficient/1
  Gain3/1 -> Gain4/1
  Gain4/1 -> Add5/1, Add4/1
  Downforce Coefficient/1 -> Gain3/1
  Gain5/1 -> Product10/2

== system Model/Drivetrain/TV Algorithm/Torque Vectoring/RB Torque Difference Calculation ==
  Desired Yaw Rate TV [deg/s] : Inport
  SWS VD Parameter 4 : Inport  Port=2
  " " : Constant  Value=1.2
  "  " : Constant  Value=13
  "   " : Constant  Value=tire_radius
  Abs : Abs  SaturateOnIntegerOverflow=off
  Compare To Constant : simulink/Logic and Bit Operations/Compare To Constant  relop===  const=1  OutDataTypeStr=boolean
  Compare To Constant1 : simulink/Logic and Bit Operations/Compare To Constant  relop===  const=2  OutDataTypeStr=boolean
  Divide3 : Product  Inputs=**
  Divide4 : Product  Inputs=*/
  Divide5 : Product  Inputs=**
  Gain : Gain  Gain=40
  Gain1 : Gain  Gain=0.5
  Gain2 : Gain  Gain=-1
  OR : Logic  Operator=OR  IconShape=distinctive  AllPortsSameDT=off  OutDataTypeStr=boolean
  Saturation : Saturate  UpperLimit=29.1  LowerLimit=0
  Switch : Switch  Criteria=u2 > Threshold  SaturateOnIntegerOverflow=off  InputSameDT=off
  Torque Difference RB [Nm] : Outport
  wires:
  Gain2/1 -> Switch/1
  Switch/1 -> Torque Difference RB [Nm]/1
  Saturation/1 -> Switch/3, Gain2/1  "Torque Difference [Nm]"
  SWS VD Parameter 4/1 -> Compare To Constant/1, Compare To Constant1/1
  Compare To Constant/1 -> OR/1
  Compare To Constant1/1 -> OR/2
  Abs/1 -> Saturation/1
  Gain1/1 -> Abs/1
  Divide4/1 -> Gain1/1
  "   "/1 -> Divide3/1
  " "/1 -> Divide5/2
  Divide5/1 -> Divide4/2
  "  "/1 -> Divide5/1
  Gain/1 -> Divide3/2
  Desired Yaw Rate TV [deg/s]/1 -> Gain/1
  Divide3/1 -> Divide4/1
  OR/1 -> Switch/2

== system Model/Drivetrain/TV Algorithm/Torque Vectoring/RB Yaw Rate Calculation ==
  SWS VD Parameter 4 : Inport
  Wheel Angle F [deg] : Inport  Port=2
  Vehicle Speed [km/h] : Inport  Port=3
  " " : Constant  Value=wheel_base
  Add : Sum
  Divide : Product  Inputs=**/
  Divide1 : Product  Inputs=**
  File Log : slrealtimeloglib/File Log  decimation=1  inputProcessing=Elements as channels (sample based)
  Square : Math  Operator=square
  Understeer Gradeint Selection : Subsystem
  Desired Yaw Rate TV RB [deg/s] : Outport
  wires:
  SWS VD Parameter 4/1 -> Understeer Gradeint Selection/1(SWS VD Parameter 4)
  Wheel Angle F [deg]/1 -> Divide/1
  Add/1 -> Divide/3
  Divide1/1 -> Add/2
  Understeer Gradeint Selection/1(Understeer Gradient) -> Divide1/2
  Square/1 -> Divide1/1
  Vehicle Speed [km/h]/1 -> Divide/2, Square/1
  Divide/1 -> Desired Yaw Rate TV RB [deg/s]/1, File Log/1  "Desired Yaw Rate TV [deg/s]"
  " "/1 -> Add/1

== system Model/Drivetrain/TV Algorithm/Torque Vectoring/Subsystem ==
  Torque After TV RL [Nm] not saturated : Inport
  SWS VD Parameter 6 : Inport  Port=2
  Torque After TV RR [Nm] not saturated : Inport  Port=3
  Bus Selector : BusSelector  OutputSignals=Torque After TV RL [Nm],Torque After TV RR [Nm]
  Merge : Merge  Inputs=11
  Switch Case : SwitchCase  CaseConditions={1,2,3,4,5,6,7,8,9,10}
  Switch Case Action Subsystem : Subsystem  TreatAsAtomicUnit=on
  Switch Case Action Subsystem1 : Subsystem  TreatAsAtomicUnit=on
  Switch Case Action Subsystem10 : Subsystem  TreatAsAtomicUnit=on
  Switch Case Action Subsystem2 : Subsystem  TreatAsAtomicUnit=on
  Switch Case Action Subsystem3 : Subsystem  TreatAsAtomicUnit=on
  Switch Case Action Subsystem4 : Subsystem  TreatAsAtomicUnit=on
  Switch Case Action Subsystem5 : Subsystem  TreatAsAtomicUnit=on
  Switch Case Action Subsystem6 : Subsystem  TreatAsAtomicUnit=on
  Switch Case Action Subsystem7 : Subsystem  TreatAsAtomicUnit=on
  Switch Case Action Subsystem8 : Subsystem  TreatAsAtomicUnit=on
  Switch Case Action Subsystem9 : Subsystem  TreatAsAtomicUnit=on
  Torque After TV RL [Nm] : Outport
  Torque After TV RR [Nm] : Outport  Port=2
  wires:
  Switch Case Action Subsystem/1(Out1) -> Merge/1
  Switch Case Action Subsystem1/1(Out1) -> Merge/2
  Switch Case Action Subsystem2/1(Out1) -> Merge/3
  Switch Case Action Subsystem3/1(Out1) -> Merge/4
  Switch Case Action Subsystem4/1(Out1) -> Merge/5
  Switch Case Action Subsystem5/1(Out1) -> Merge/6
  Switch Case Action Subsystem6/1(Out1) -> Merge/7
  Switch Case Action Subsystem7/1(Out1) -> Merge/8
  Switch Case Action Subsystem8/1(Out1) -> Merge/9
  Switch Case Action Subsystem9/1(Out1) -> Merge/10
  Switch Case Action Subsystem10/1(Out1) -> Merge/11
  SWS VD Parameter 6/1 -> Switch Case/1
  Switch Case/1 -> Switch Case Action Subsystem/Action
  Switch Case/2 -> Switch Case Action Subsystem1/Action
  Switch Case/3 -> Switch Case Action Subsystem2/Action
  Switch Case/4 -> Switch Case Action Subsystem3/Action
  Switch Case/5 -> Switch Case Action Subsystem4/Action
  Switch Case/6 -> Switch Case Action Subsystem5/Action
  Switch Case/7 -> Switch Case Action Subsystem6/Action
  Switch Case/8 -> Switch Case Action Subsystem7/Action
  Switch Case/9 -> Switch Case Action Subsystem8/Action
  Switch Case/10 -> Switch Case Action Subsystem9/Action
  Switch Case/11 -> Switch Case Action Subsystem10/Action
  Torque After TV RL [Nm] not saturated/1 -> Switch Case Action Subsystem10/1(Torque After TV RL [Nm] not saturated), Switch Case Action Subsystem9/1(Torque After TV RL [Nm] not saturated), Switch Case Action Subsystem8/1(Torque After TV RL [Nm] not saturated), Switch Case Action Subsystem7/1(Torque After TV RL [Nm] not saturated), Switch Case Action Subsystem6/1(Torque After TV RL [Nm] not saturated), Switch Case Action Subsystem5/1(Torque After TV RL [Nm] not saturated), Switch Case Action Subsystem3/1(Torque After TV RL [Nm] not saturated), Switch Case Action Subsystem1/1(Torque After TV RL [Nm] not saturated), Switch Case Action Subsystem/1(Torque After TV RL [Nm] not saturated), Switch Case Action Subsystem2/1(Torque After TV RL [Nm] not saturated), Switch Case Action Subsystem4/1(Torque After TV RL [Nm] not saturated)
  Torque After TV RR [Nm] not saturated/1 -> Switch Case Action Subsystem/2(Torque After TV RR [Nm] not saturated), Switch Case Action Subsystem1/2(Torque After TV RR [Nm] not saturated), Switch Case Action Subsystem2/2(Torque After TV RR [Nm] not saturated), Switch Case Action Subsystem3/2(Torque After TV RR [Nm] not saturated), Switch Case Action Subsystem4/2(Torque After TV RR [Nm] not saturated), Switch Case Action Subsystem5/2(Torque After TV RR [Nm] not saturated), Switch Case Action Subsystem6/2(Torque After TV RR [Nm] not saturated), Switch Case Action Subsystem7/2(Torque After TV RR [Nm] not saturated), Switch Case Action Subsystem8/2(Torque After TV RR [Nm] not saturated), Switch Case Action Subsystem9/2(Torque After TV RR [Nm] not saturated), Switch Case Action Subsystem10/2(Torque After TV RR [Nm] not saturated)
  Merge/1 -> Bus Selector/1
  Bus Selector/1 -> Torque After TV RL [Nm]/1  "<Torque After TV RL [Nm]>"
  Bus Selector/2 -> Torque After TV RR [Nm]/1  "<Torque After TV RR [Nm]>"

== system Model/Drivetrain/TV Algorithm/Torque Vectoring/Subsystem1 ==
  Torque After TV RL [Nm] not saturated : Inport
  Torque After TV RR [Nm] not saturated : Inport  Port=2
  SWS VD Parameter 6 : Inport  Port=3
  Bus Selector : BusSelector  OutputSignals=Torque After TV RL [Nm],Torque After TV RR [Nm]
  Merge : Merge  Inputs=11
  Switch Case : SwitchCase  CaseConditions={1,2,3,4,5,6,7,8,9,10}
  Switch Case Action Subsystem : Subsystem  TreatAsAtomicUnit=on
  Switch Case Action Subsystem1 : Subsystem  TreatAsAtomicUnit=on
  Switch Case Action Subsystem10 : Subsystem  TreatAsAtomicUnit=on
  Switch Case Action Subsystem2 : Subsystem  TreatAsAtomicUnit=on
  Switch Case Action Subsystem3 : Subsystem  TreatAsAtomicUnit=on
  Switch Case Action Subsystem4 : Subsystem  TreatAsAtomicUnit=on
  Switch Case Action Subsystem5 : Subsystem  TreatAsAtomicUnit=on
  Switch Case Action Subsystem6 : Subsystem  TreatAsAtomicUnit=on
  Switch Case Action Subsystem7 : Subsystem  TreatAsAtomicUnit=on
  Switch Case Action Subsystem8 : Subsystem  TreatAsAtomicUnit=on
  Switch Case Action Subsystem9 : Subsystem  TreatAsAtomicUnit=on
  Torque After TV RL [Nm] : Outport
  Torque After TV RR [Nm] : Outport  Port=2
  wires:
  Bus Selector/2 -> Torque After TV RR [Nm]/1  "<Torque After TV RR [Nm]>"
  Bus Selector/1 -> Torque After TV RL [Nm]/1  "<Torque After TV RL [Nm]>"
  Merge/1 -> Bus Selector/1
  Torque After TV RR [Nm] not saturated/1 -> Switch Case Action Subsystem10/2(Torque After TV RR [Nm] not saturated), Switch Case Action Subsystem9/2(Torque After TV RR [Nm] not saturated), Switch Case Action Subsystem8/2(Torque After TV RR [Nm] not saturated), Switch Case Action Subsystem7/2(Torque After TV RR [Nm] not saturated), Switch Case Action Subsystem6/2(Torque After TV RR [Nm] not saturated), Switch Case Action Subsystem5/2(Torque After TV RR [Nm] not saturated), Switch Case Action Subsystem4/2(Torque After TV RR [Nm] not saturated), Switch Case Action Subsystem3/2(Torque After TV RR [Nm] not saturated), Switch Case Action Subsystem2/2(Torque After TV RR [Nm] not saturated), Switch Case Action Subsystem1/2(Torque After TV RR [Nm] not saturated), Switch Case Action Subsystem/2(Torque After TV RR [Nm] not saturated)
  Torque After TV RL [Nm] not saturated/1 -> Switch Case Action Subsystem4/1(Torque After TV RL [Nm] not saturated), Switch Case Action Subsystem2/1(Torque After TV RL [Nm] not saturated), Switch Case Action Subsystem/1(Torque After TV RL [Nm] not saturated), Switch Case Action Subsystem1/1(Torque After TV RL [Nm] not saturated), Switch Case Action Subsystem3/1(Torque After TV RL [Nm] not saturated), Switch Case Action Subsystem5/1(Torque After TV RL [Nm] not saturated), Switch Case Action Subsystem6/1(Torque After TV RL [Nm] not saturated), Switch Case Action Subsystem7/1(Torque After TV RL [Nm] not saturated), Switch Case Action Subsystem8/1(Torque After TV RL [Nm] not saturated), Switch Case Action Subsystem9/1(Torque After TV RL [Nm] not saturated), Switch Case Action Subsystem10/1(Torque After TV RL [Nm] not saturated)
  Switch Case/11 -> Switch Case Action Subsystem10/Action
  Switch Case/10 -> Switch Case Action Subsystem9/Action
  Switch Case/9 -> Switch Case Action Subsystem8/Action
  Switch Case/8 -> Switch Case Action Subsystem7/Action
  Switch Case/7 -> Switch Case Action Subsystem6/Action
  Switch Case/6 -> Switch Case Action Subsystem5/Action
  Switch Case/5 -> Switch Case Action Subsystem4/Action
  Switch Case/4 -> Switch Case Action Subsystem3/Action
  Switch Case/3 -> Switch Case Action Subsystem2/Action
  Switch Case/2 -> Switch Case Action Subsystem1/Action
  Switch Case/1 -> Switch Case Action Subsystem/Action
  SWS VD Parameter 6/1 -> Switch Case/1
  Switch Case Action Subsystem10/1(Out1) -> Merge/11
  Switch Case Action Subsystem9/1(Out1) -> Merge/10
  Switch Case Action Subsystem8/1(Out1) -> Merge/9
  Switch Case Action Subsystem7/1(Out1) -> Merge/8
  Switch Case Action Subsystem6/1(Out1) -> Merge/7
  Switch Case Action Subsystem5/1(Out1) -> Merge/6
  Switch Case Action Subsystem4/1(Out1) -> Merge/5
  Switch Case Action Subsystem3/1(Out1) -> Merge/4
  Switch Case Action Subsystem2/1(Out1) -> Merge/3
  Switch Case Action Subsystem1/1(Out1) -> Merge/2
  Switch Case Action Subsystem/1(Out1) -> Merge/1

== system Model/Drivetrain/TV Algorithm/Torque Vectoring/Subsystem2 ==
  Brakes : Inport
  In3 : Inport  Port=2
  AND2 : Logic  IconShape=distinctive  AllPortsSameDT=off  OutDataTypeStr=boolean
  Bus Selector : BusSelector  OutputSignals=Front,Rear
  Compare To Constant3 : simulink/Logic and Bit Operations/Compare To Constant  relop=>=  const=5  OutDataTypeStr=boolean
  Compare To Constant4 : simulink/Logic and Bit Operations/Compare To Constant  relop=>=  const=5  OutDataTypeStr=boolean
  OR : Logic  Operator=OR  IconShape=distinctive  AllPortsSameDT=off  OutDataTypeStr=boolean
  Regen Braking Check : Outport
  wires:
  AND2/1 -> Regen Braking Check/1  "Regen Braking Check"
  Compare To Constant3/1 -> OR/2
  OR/1 -> AND2/1
  Compare To Constant4/1 -> OR/1
  In3/1 -> AND2/2
  Bus Selector/1 -> Compare To Constant4/1  "<Front>"
  Brakes/1 -> Bus Selector/1
  Bus Selector/2 -> Compare To Constant3/1  "<Rear>"

== system Model/Drivetrain/TV Algorithm/Torque Vectoring/TV Activation ==
  Wheel Angle F [deg] : Inport
  Vehicle Speed [km/h] : Inport  Port=2
  SWS VD Setup 3 : Inport  Port=3
  Regen Braking Check : Inport  Port=4
  R2D Status : Inport  Port=5
  AND : Logic  Inputs=5  IconShape=distinctive  AllPortsSameDT=off  OutDataTypeStr=boolean
  Compare To Constant : simulink/Logic and Bit Operations/Compare To Constant  relop=>=  const=3  OutDataTypeStr=boolean
  Compare To Constant1 : simulink/Logic and Bit Operations/Compare To Constant  relop=<=  const=-3  OutDataTypeStr=boolean
  Compare To Constant2 : simulink/Logic and Bit Operations/Compare To Constant  relop=>  const=-1  OutDataTypeStr=boolean
  NOT : Logic  Operator=NOT  IconShape=distinctive  AllPortsSameDT=off  OutDataTypeStr=boolean
  OR1 : Logic  Operator=OR  IconShape=distinctive  AllPortsSameDT=off  OutDataTypeStr=boolean
  TV Active : Outport
  wires:
  AND/1 -> TV Active/1
  R2D Status/1 -> AND/2
  SWS VD Setup 3/1 -> AND/1
  Compare To Constant1/1 -> OR1/2
  Compare To Constant/1 -> OR1/1
  Wheel Angle F [deg]/1 -> Compare To Constant/1, Compare To Constant1/1
  Vehicle Speed [km/h]/1 -> Compare To Constant2/1
  Compare To Constant2/1 -> AND/3
  OR1/1 -> AND/4
  Regen Braking Check/1 -> NOT/1
  NOT/1 -> AND/5

== system Model/Drivetrain/TV Algorithm/Torque Vectoring/TV RB Activation ==
  R2D Status : Inport
  Regen Braking Check : Inport  Port=2
  Vehicle Speed [km/h] : Inport  Port=3
  SWS VD Setup 4 : Inport  Port=4
  Wheel Angle F [deg] : Inport  Port=5
  AND : Logic  Inputs=5  IconShape=distinctive  AllPortsSameDT=off  OutDataTypeStr=boolean
  Compare To Constant : simulink/Logic and Bit Operations/Compare To Constant  relop=>=  const=3  OutDataTypeStr=boolean
  Compare To Constant1 : simulink/Logic and Bit Operations/Compare To Constant  relop=<=  const=-3  OutDataTypeStr=boolean
  Compare To Constant2 : simulink/Logic and Bit Operations/Compare To Constant  relop=>  const=10  OutDataTypeStr=boolean
  OR1 : Logic  Operator=OR  IconShape=distinctive  AllPortsSameDT=off  OutDataTypeStr=boolean
  TV RB Active : Outport
  wires:
  OR1/1 -> AND/4
  Wheel Angle F [deg]/1 -> Compare To Constant1/1, Compare To Constant/1
  Compare To Constant/1 -> OR1/1
  Compare To Constant1/1 -> OR1/2
  SWS VD Setup 4/1 -> AND/1
  R2D Status/1 -> AND/2
  AND/1 -> TV RB Active/1
  Vehicle Speed [km/h]/1 -> Compare To Constant2/1
  Compare To Constant2/1 -> AND/3
  Regen Braking Check/1 -> AND/5

== system Model/Drivetrain/TV Algorithm/Torque Vectoring/Torque Difference Calculation ==
  Desired Yaw Rate TV [deg/s] : Inport
  SWS VD Setup 15 : Inport  Port=2
  SWS VD Parameter 3 : Inport  Port=3
  " " : Constant  Value=1.2
  "  " : Constant  Value=13
  "   " : Constant  Value=tire_radius
  AND : Logic  IconShape=distinctive  AllPortsSameDT=off  OutDataTypeStr=boolean
  Abs : Abs  SaturateOnIntegerOverflow=off
  Compare To Constant : simulink/Logic and Bit Operations/Compare To Constant  relop===  const=1  OutDataTypeStr=boolean
  Compare To Constant1 : simulink/Logic and Bit Operations/Compare To Constant  relop===  const=2  OutDataTypeStr=boolean
  Compare To Constant2 : simulink/Logic and Bit Operations/Compare To Constant  relop===  const=0  OutDataTypeStr=boolean
  Divide3 : Product  Inputs=**
  Divide4 : Product  Inputs=*/
  Divide5 : Product  Inputs=**
  Gain : Gain  Gain=40
  Gain1 : Gain  Gain=0.5
  Gain2 : Gain  Gain=-1
  OR : Logic  Operator=OR  IconShape=distinctive  AllPortsSameDT=off  OutDataTypeStr=boolean
  Saturation : Saturate  UpperLimit=Torque_limit_max  LowerLimit=0
  Switch : Switch  Criteria=u2 > Threshold  SaturateOnIntegerOverflow=off  InputSameDT=off
  Torque Difference [Nm] : Outport
  wires:
  Divide3/1 -> Divide4/1
  Desired Yaw Rate TV [deg/s]/1 -> Gain/1
  Gain/1 -> Divide3/2
  "  "/1 -> Divide5/1
  Divide5/1 -> Divide4/2
  " "/1 -> Divide5/2
  "   "/1 -> Divide3/1
  Divide4/1 -> Gain1/1
  Gain1/1 -> Abs/1
  Abs/1 -> Saturation/1
  Compare To Constant1/1 -> OR/2
  Compare To Constant/1 -> OR/1
  SWS VD Parameter 3/1 -> Compare To Constant1/1, Compare To Constant/1
  Saturation/1 -> Gain2/1, Switch/3  "Torque Difference [Nm]"
  Switch/1 -> Torque Difference [Nm]/1
  Gain2/1 -> Switch/1
  OR/1 -> AND/1
  SWS VD Setup 15/1 -> Compare To Constant2/1
  AND/1 -> Switch/2
  Compare To Constant2/1 -> AND/2
